simulink model "encoder1"  (R2022b)
settings: Solver=VariableStepAuto  StartTime=0.0  StopTime=200  RelTol=1e-3
libraries: simulink x8, spsSampleandHoldLib x2
settings Model: Creator=mluser  LastModifiedBy=mluser

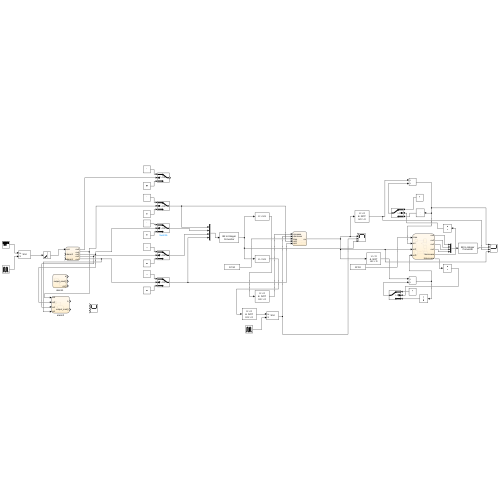
[thumbnail: Simulink's stored preview of the top-level diagram]
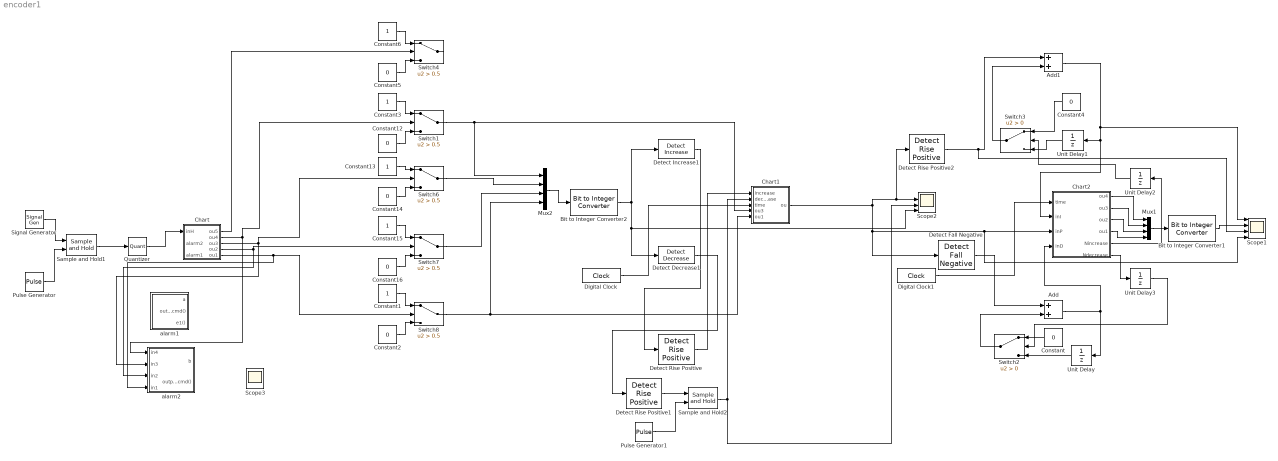
== system encoder1 ==
  Add : Sum
  Add1 : Sum
  Bit to Integer Converter1 : simulink/Logic and Bit Operations/Bit to Integer Converter  nbits=4  bitOrder=MSB first  signedOutputValues=Unsigned  outDtype=Inherit via internal rule  outDtypeSigned=Inherit via internal rule
  Bit to Integer Converter2 : simulink/Logic and Bit Operations/Bit to Integer Converter  nbits=4  bitOrder=MSB first  signedOutputValues=Unsigned  outDtype=Inherit via internal rule  outDtypeSigned=Inherit via internal rule
  Chart : Stateflow chart  TreatAsAtomicUnit=on
      settings: PortSchema="{\"entries\":[{\"content\":{\"sides\":[{\"content\":{\"connectorIds\":[\"In1\",\"In2\",\"In3\"]},\"type\":\"ConnectorPlacement.EquallySpacedRectSide\",\"uuid\":\"aaeedc4a-65ef-4d8f-ba01-1ddc4e011816\"},{\"content\":{\"connectorIds\":[\"Out5\",\"Out2\",\"Out1\",\"Out3\",\"Out4\"],\"side\":\"RIGHT\"},\"type\":\"ConnectorPlacement.EquallySpacedRectSide\",\"uuid\":\"bfc75945-f598-4b29-99c0-df6bb3f156b5\"},{\"content\":{\"connectorIds\":[],\"side\":\"TOP\"},\"type\":\"ConnectorPlacement.EquallySpacedRectSide\",\"uuid\":\"e78d9c07-753c-4a5b-aa63-095c584c660c\"}]},\"type\":\"ConnectorPlacement.EquallySpacedConnector\",\"uuid\":\"f46ef6be-e67f-4bb7-838b-d108f8d3e6f5\"}],\"packageUris\":[\"http://schema.mathworks.com/mf0/Connector/R2020b\"],\"version\":\"1.0\"}"
  Chart1 : Stateflow chart  TreatAsAtomicUnit=on
  Chart2 : Stateflow chart  TreatAsAtomicUnit=on
      settings: PortSchema="{\"entries\":[{\"content\":{\"sides\":[{\"content\":{\"connectorIds\":[\"In1\",\"In4\",\"In3\",\"In2\"]},\"type\":\"ConnectorPlacement.EquallySpacedRectSide\",\"uuid\":\"2f71a724-cbde-41d0-addd-3c968d2e9507\"},{\"content\":{\"connectorIds\":[\"Out2\",\"Out3\",\"Out1\",\"Out4\",\"Out5\",\"Out6\"],\"side\":\"RIGHT\"},\"type\":\"ConnectorPlacement.EquallySpacedRectSide\",\"uuid\":\"fd511e75-9748-4994-ae8b-80feb2a63518\"},{\"content\":{\"connectorIds\":[],\"side\":\"TOP\"},\"type\":\"ConnectorPlacement.EquallySpacedRectSide\",\"uuid\":\"1de50c17-1645-4694-9a4a-35d7a7d0bb59\"}]},\"type\":\"ConnectorPlacement.EquallySpacedConnector\",\"uuid\":\"36ccd1b3-f5fe-461c-b238-a087658ad9ff\"}],\"packageUris\":[\"http://schema.mathworks.com/mf0/Connector/R2020b\"],\"version\":\"1.0\"}"
  Constant{,2,4..5,12,14,16} (7 alike) : Constant  Value=0
  Constant{1,3,6,13,15} (5 alike) : Constant
  Detect Decrease1 : simulink/Logic and Bit Operations/Detect Decrease  vinit=0.0  OutDataTypeStr=boolean
  Detect Increase1 : simulink/Logic and Bit Operations/Detect Increase  vinit=0.0  OutDataTypeStr=boolean
  Detect Fall Negative : simulink/Logic and Bit Operations/Detect Fall Negative  vinit=0  OutDataTypeStr=boolean
  Detect Rise Positive : simulink/Logic and Bit Operations/Detect Rise Positive  vinit=0  OutDataTypeStr=boolean
  Detect Rise Positive1 : simulink/Logic and Bit Operations/Detect Rise Positive  vinit=0  OutDataTypeStr=boolean
  Detect Rise Positive2 : simulink/Logic and Bit Operations/Detect Rise Positive  vinit=0  OutDataTypeStr=boolean
  Digital Clock : DigitalClock  SampleTime=0.01
  Digital Clock1 : DigitalClock  SampleTime=0.01
  Mux1 : Mux
  Mux2 : Mux
  Pulse Generator : DiscretePulseGenerator  PulseType=Time based  Period=0.01  PulseWidth=5  PhaseDelay=0.1
  Pulse Generator1 : DiscretePulseGenerator  PulseType=Time based  Period=0.01  PulseWidth=5
  Quantizer : Quantizer
  Sample and Hold1 : spsSampleandHoldLib/Sample and Hold  ic=0  Ts=0.1
  Sample and Hold2 : spsSampleandHoldLib/Sample and Hold  ic=0  Ts=0.01
  Scope1 : Scope  NumInputPorts=4
  Scope2 : Scope  NumInputPorts=4
  Scope3 : Scope  NumInputPorts=4
  Signal Generator : SignalGenerator  Amplitude=40  Frequency=0.02  Units=rad/sec
  Switch{1,4,6..8} (5 alike) : Switch  Criteria=u2 > Threshold  Threshold=0.5  SaturateOnIntegerOverflow=off  InputSameDT=off
  Switch2 : Switch  Criteria=u2 > Threshold  SaturateOnIntegerOverflow=off  InputSameDT=off
  Switch3 : Switch  Criteria=u2 > Threshold  SaturateOnIntegerOverflow=off  InputSameDT=off
  Unit Delay{,1..3} (4 alike) : UnitDelay  SampleTime=-1  HasFrameUpgradeWarning=on
  alarm1 : Stateflow chart  TreatAsAtomicUnit=on
  alarm2 : Stateflow chart  TreatAsAtomicUnit=on
      settings: PortSchema="{\"entries\":[{\"content\":{\"sides\":[{\"content\":{\"connectorIds\":[\"In4\",\"In1\",\"In2\",\"In3\"]},\"type\":\"ConnectorPlacement.EquallySpacedRectSide\",\"uuid\":\"c2a534fa-eabb-4b72-8afe-e20b3966ee5f\"},{\"content\":{\"connectorIds\":[\"Out1\",\"Out2\"],\"side\":\"RIGHT\"},\"type\":\"ConnectorPlacement.EquallySpacedRectSide\",\"uuid\":\"3d761f63-15fa-4251-9a6b-ba3c44659912\"},{\"content\":{\"connectorIds\":[],\"side\":\"TOP\"},\"type\":\"ConnectorPlacement.EquallySpacedRectSide\",\"uuid\":\"cb0b1e27-d1c1-4ffa-8e03-dfec8c9ecea8\"}]},\"type\":\"ConnectorPlacement.EquallySpacedConnector\",\"uuid\":\"863d097b-aacc-4bdd-a8c2-65eaa9078137\"}],\"packageUris\":[\"http://schema.mathworks.com/mf0/Connector/R2020b\"],\"version\":\"1.0\"}"
  wires:
  Pulse Generator/1 -> Sample and Hold1/2
  Signal Generator/1 -> Sample and Hold1/1
  Sample and Hold1/1 -> Quantizer/1
  Quantizer/1 -> Chart/1(inH)
  Constant3/1 -> Switch1/1
  Constant14/1 -> Switch6/3
  Constant15/1 -> Switch7/1
  Constant13/1 -> Switch6/1
  Constant16/1 -> Switch7/3
  Chart/3(ou2) -> Switch7/2, alarm2/2(in2)
  Constant12/1 -> Switch1/3
  Switch1/1 -> Mux2/1, Chart1/4(ou3)
  Constant1/1 -> Switch8/1
  Constant2/1 -> Switch8/3
  Chart/4(ou1) -> alarm2/3(in1), Switch8/2
  Mux2/1 -> Bit to Integer Converter2/1
  Bit to Integer Converter2/1 -> Detect Decrease1/1, Scope2/4, Detect Increase1/1
  Detect Increase1/1 -> Detect Rise Positive/1
  Detect Decrease1/1 -> Detect Rise Positive1/1
  Digital Clock/1 -> Chart1/3(time)
  Digital Clock1/1 -> Chart2/1(time)
  Chart2/4(ou1) -> Mux1/4
  Chart2/1(ou2) -> Mux1/3
  Chart2/3(ou3) -> Mux1/2
  Chart2/2(ou4) -> Mux1/1
  Mux1/1 -> Bit to Integer Converter1/1
  Detect Rise Positive/1 -> Chart1/1(increase)
  Detect Rise Positive1/1 -> Sample and Hold2/1
  Sample and Hold2/1 -> Scope2/3, Chart1/2(decrease)
  Pulse Generator1/1 -> Sample and Hold2/2
  Add/1 -> Chart2/2(inD), Unit Delay/1
  Detect Fall Negative/1 -> Add/1
  Constant/1 -> Switch2/1
  Unit Delay/1 -> Switch2/3
  Switch2/1 -> Add/2
  Unit Delay1/1 -> Switch3/3
  Constant4/1 -> Switch3/1
  Switch3/1 -> Add1/2
  Chart2/5(Nincrease) -> Unit Delay2/1
  Unit Delay2/1 -> Switch3/2
  Chart2/6(Ndecrease) -> Unit Delay3/1
  Unit Delay3/1 -> Switch2/2
  Add1/1 -> Scope1/1, Chart2/4(inI), Unit Delay1/1
  Detect Rise Positive2/1 -> Scope1/3, Add1/1
  Chart1/1(ou) -> Detect Fall Negative/1, Scope1/4, Chart2/3(inP), Detect Rise Positive2/1, Scope2/2
  Bit to Integer Converter1/1 -> Scope1/2
  Chart/1(ou3) -> Switch6/2, alarm2/1(in3)
  Chart/2(ou4) -> Switch1/2, alarm2/4(in4)
  Constant6/1 -> Switch4/1
  Constant5/1 -> Switch4/3
  Chart/5(ou5) -> Switch4/2
  Switch8/1 -> Mux2/4, Chart1/5(ou1)
  Switch6/1 -> Mux2/2
  Switch7/1 -> Mux2/3

== stateflow chart encoder1/Chart1 ==
  (default) -> (junction 3)
  (junction 3) -> (junction 28) [order 2] : [increase==1&&time>0]
  (junction 28) -> (junction 44) : {ou=1;}
  (junction 3) -> (junction 10) [order 1]
  (junction 44) -> (junction 43)
  (junction 10) -> (junction 8) [order 1] : [decrease==1&&time>0]
  (junction 8) -> (junction 43) : {ou=-1;}
  (junction 10) -> (junction 71) [order 2]
  (junction 43) -> (junction 72)
  (junction 71) -> (junction 73) [order 1] : [time==0&&ou3==1]
  (junction 73) -> (junction 72) : {ou=1;}
  (junction 71) -> (junction 78) [order 2]
  (junction 72) -> (junction 80)
  (junction 78) -> (junction 79) [order 1] : [time==0&&ou1==0]
  (junction 79) -> (junction 80) : {ou=-1;}
  (junction 78) -> (junction 90) [order 2]
  (junction 80) -> (junction 88)
  (junction 89) -> (junction 88) : {ou=0}
  (junction 90) -> (junction 89) : [increase==0&&decrease==0]
  data: increase input; decrease input; ou output; time input; ou3 input; ou1 input

== stateflow chart encoder1/Chart2 ==
  state state1
    entry:
    ou1=0;ou2=0;
    ou3=0;ou4=0;
    Ndecrease=0;
    Nincrease=0;
  state initial
    entry:
    Ndecrease=1;
    Nincrease=1;
  state state2
    entry:
    ou1=1;ou2=1;
    ou3=0;ou4=0;
    Ndecrease=0;
    Nincrease=0;
  state state4
    entry:
    ou1=1;ou2=1;
    ou3=1;ou4=1;
    Ndecrease=0;
    Nincrease=0;
  state state3
    entry:
    ou1=1;ou2=1;
    ou3=1;ou4=0;
    Nincrease=0;
    Ndecrease=0;
  (default) -> initial
  initial -> state1 [order 2] : [time<1&&inP==1]
      | {Ndecrease=0;
      | Nincrease=0;}
  initial -> state4 [order 1] : [time<1&&inP==-1]
  state1 -> state2 : [time>=1&&inP==1&&inI==1]
  (junction 120) -> state1 : {Ndecrease=1;
      | Nincrease=1;}
  state2 -> (junction 120) [order 1] : [time>=1&&inP==-1&&inD==3]
  state3 -> state2 [order 2] : [time>=1&&inP==-1&&inD==2]
  state2 -> state3 [order 2] : [time>=1&&inP==1&&inI==2]
  state3 -> (junction 124) [order 1] : [time>=1&&inP==1&&inI==3]
  (junction 124) -> state4 : {Ndecrease=1;
      | Nincrease=1;}
  state4 -> state3 : [time>=1&&inP==-1&&inD==1]
  data: time input; inD input; inP input; inI input; ou2 output; ou4 output; ou3 output; ou1 output; Nincrease output; Ndecrease output

== stateflow chart encoder1/Chart ==
  (default) -> (junction 3) : {ou1=0;
      | ou2=0;
      | ou3=0;
      | ou4=0;
      | ou5=0;
      | }
  (junction 3) -> (junction 28) [order 2] : [inH==0]
  (junction 28) -> (junction 44) : {ou1=0;ou2=0;ou3=0;ou4=0;}
  (junction 3) -> (junction 10) [order 1]
  (junction 44) -> (junction 43)
  (junction 10) -> (junction 8) [order 1] : [inH<=10]
  (junction 8) -> (junction 43) : {ou1=1;ou2=0;ou3=0;ou4=0;}
  (junction 10) -> (junction 12) [order 2]
  (junction 43) -> (junction 42)
  (junction 16) -> (junction 42) : {ou1=1;ou2=1;ou3=0;ou4=0;}
  (junction 12) -> (junction 16) [order 1] : [inH>10&&inH<=20]
  (junction 42) -> (junction 41)
  (junction 12) -> (junction 19) [order 2]
  (junction 19) -> (junction 18) [order 1] : [inH>20&&inH<=30]
  (junction 18) -> (junction 41) : {ou1=1;ou2=1;ou3=1;ou4=0;}
  (junction 41) -> (junction 63)
  (junction 19) -> (junction 61) [order 2]
  (junction 61) -> (junction 62) [order 1] : [inH>30]
  (junction 62) -> (junction 63) : {ou1=1;ou2=1;ou3=1;ou4=1;}
  (junction 61) -> (junction 69) [order 2]
  (junction 63) -> (junction 71)
  (junction 69) -> (junction 70) [order 1] : [alarm1==1]
  (junction 70) -> (junction 71) : {ou1=0;ou2=0;ou3=0;ou4=1;ou5=0;}
  (junction 69) -> (junction 76) [order 2]
  (junction 71) -> (junction 78)
  (junction 76) -> (junction 77) : [alarm2==1]
  (junction 77) -> (junction 78) : {ou1=0;ou2=0;ou3=0;ou4=0;ou5=1;}
  data: ou3 output; ou4 output; ou2 output; ou1 output; inH input; alarm2 input; alarm1 input; ou5 output

== stateflow chart encoder1/alarm1 ==
  state alarm1
    du:a=0;
  state end
    en:
    send(e1);
    du:a=1;
  (default) -> alarm1
  alarm1 -> end : after(100,sec)
  end -> alarm1 : after(2,sec)
  data: a output
  events: output_cmd output FUNCTION_CALL_EVENT; e1 output FUNCTION_CALL_EVENT

== stateflow chart encoder1/alarm2 ==
  state alarm2
    du:
    b=0;
  state end
    en:
    send(output_cmd);
    du:
    b=1;
  (default) -> alarm2
  alarm2 -> (junction 75) [order 1] : [in4==1&&in3==1&&in2==1&&in1==1]
  (junction 75) -> end : after(20,sec)
  alarm2 -> end [order 2] : after(2,sec)
  data: in3 input; in2 input; in1 input; in4 input; b output
  events: output_cmd output FUNCTION_CALL_EVENT
